simulink model "nmsRR"  (R2021a)
settings: Solver=ode15s  StartTime=0.0  StopTime=t  MaxStep=1e-2  RelTol=1e-2
StartFcn:
  | tic
StopFcn:
  | toc
  | 
  | 
  | %if GimbalLockFlag
  |  % fprintf(2, 'Almost reached Gimbal Lock of IMU. Simulation stopped.\n')
  | %end
  | 
  | %fprintf('Elapsed time: %4.2f sec (%4.2f%% realtime)\n', a, tout(end)/a*100)
undefined symbols (not defined in the file): Balance02, Balance13, BalanceTrunk, BasisStim, CompensateSwing, CompliantLeg, FlexAnkle, Ground, ICs, init_des_left, init_des_right, init_l_left, init_l_right, init_q_del, init_sensor_body, init_sensor_world, init_v_left, init_v_right, LateralControl, mParams, PreventKneeOverextension, StepDur, Target02, Target13, theta0, X, Y, Z
libraries: simulink_extras x133, nesl_utility x105, sm_lib x88, simulink x72, robotcorelib x5, dspinverses x5, dspswit3 x2, vrlib x2, robotmaniplib x1
(part 7 of 8)

== system nmsRR/Body and Contact Model/Vestibular System/Align Axis/Compute Saggital Rotation ==
  Hip Position Left [m] : Inport
  Hip Position Right [m] : Inport  Port=2
  Trunk Position [m] : Inport  Port=3
  Constant : Constant  Value=[0 1 0]
  Constant1 : Constant
  Constant2 : Constant  Value=-1
  Dot Product : DotProduct  InputSameDT=on  OutDataTypeStr=Inherit: Inherit via internal rule
  Gain : Gain  Gain=[0.5 0.5 0]
  Gain1 : Gain  Gain=[1 1 0]
  Minus : Sum
  Minus1 : Sum  Inputs=+-
  Product : Product
  Selector : Selector  InputPortWidth=3  IndexOptions=Index vector (dialog)  Indices=[1]  OutputSizes=1
  Switch : Switch  Criteria=u2 > Threshold
  Trigonometric Function : Trigonometry  Operator=acos
  compute angle witth y axis5 : Subsystem  Commented=on
  normalize : Subsystem
  Saggital Rotation : Outport
  wires:
  Hip Position Right [m]/1 -> Minus/1
  Trigonometric Function/1 -> Product/2
  Constant/1 -> Dot Product/1
  Dot Product/1 -> Trigonometric Function/1
  Hip Position Left [m]/1 -> Minus/2
  Minus/1 -> Gain/1
  Gain/1 -> Minus1/2
  Trunk Position [m]/1 -> Gain1/1
  Minus1/1 -> normalize/1(vector)
  Selector/1 -> Switch/2
  normalize/1(norm) -> compute angle witth y axis5/1(vector), Dot Product/2, Selector/1
  Constant1/1 -> Switch/3
  Constant2/1 -> Switch/1
  Switch/1 -> Product/1
  Product/1 -> Saggital Rotation/1
  Gain1/1 -> Minus1/1

== system nmsRR/Body and Contact Model/Vestibular System/R Movement direction/normalize ==
  vector : Inport
  Divide : Product  Inputs=*/  RndMeth=Zero  SaturateOnIntegerOverflow=on
  Matrix Sum : Sum  Inputs=+
  Sqrt : Sqrt  SaturateOnIntegerOverflow=on
  Square : Math  Operator=square  SaturateOnIntegerOverflow=on
  norm : Outport
  wires:
  vector/1 -> Square/1, Divide/1
  Matrix Sum/1 -> Sqrt/1
  Divide/1 -> norm/1
  Sqrt/1 -> Divide/2
  Square/1 -> Matrix Sum/1

== system nmsRR/Muscle Actuation Layer/Muscles Left/Muscle Dynamics (Vectorized)1/BE force-length relation ==
  note: Buffer Elasticity BE
  lce [lopt] : Inport
  Constant1 : Constant  Value=1-mParams.muscles.w
  Math Function : Math  Operator=square  SignedPower=on  SaturateOnIntegerOverflow=on
  Sum4 : Sum  Inputs=|+-  InputSameDT=on  SaturateOnIntegerOverflow=on  OutDataTypeStr=Inherit: Same as first input
  buffer engaged? : simulink/Logic and Bit Operations/Compare To Zero  relop=<  OutDataTypeStr=boolean  ZeroCross=off
  force of buffer elasticity : Product  Inputs=**
  reference strain [lslack] : Constant  Value=mParams.muscles.w/2
  relative strain : Product  Inputs=*/
  fbe [Fmax] : Outport  VectorParamsAs1DForOutWhenUnconnected=off
  wires:
  force of buffer elasticity/1 -> fbe [Fmax]/1
  Math Function/1 -> force of buffer elasticity/2
  buffer engaged?/1 -> force of buffer elasticity/1
  Constant1/1 -> Sum4/2
  Sum4/1 -> relative strain/1, buffer engaged?/1
  reference strain [lslack]/1 -> relative strain/2
  relative strain/1 -> Math Function/1
  lce [lopt]/1 -> Sum4/1

== system nmsRR/Muscle Actuation Layer/Muscles Left/Muscle Dynamics (Vectorized)1/CE force-length relation ==
  note: CE Force-Length Relationship
  lce [lopt] : Inport
  Abs : Abs
  Constant1 : Constant
  Constant2 : Constant  Value=3
  Gain : Gain  Gain=log(mParams.muscles.c)
  Math Function : Math  SignedPower=on  SaturateOnIntegerOverflow=on
  Math Function1 : Math  Operator=pow  SignedPower=on  SaturateOnIntegerOverflow=on
  Sum4 : Sum  Inputs=|+-  InputSameDT=on  SaturateOnIntegerOverflow=on  OutDataTypeStr=Inherit: Same as first input
  normalized position : Product  Inputs=*/
  relative width : Constant  Value=mParams.muscles.w
  fce [Fmax] : Outport  VectorParamsAs1DForOutWhenUnconnected=off
  wires:
  Math Function/1 -> fce [Fmax]/1
  Gain/1 -> Math Function/1
  Math Function1/1 -> Gain/1
  Constant2/1 -> Math Function1/2
  normalized position/1 -> Math Function1/1
  Abs/1 -> normalized position/1
  Sum4/1 -> Abs/1
  Constant1/1 -> Sum4/2
  relative width/1 -> normalized position/2
  lce [lopt]/1 -> Sum4/1

== system nmsRR/Muscle Actuation Layer/Muscles Left/Muscle Dynamics (Vectorized)1/CE inverse force-velocity relation ==
  note: CE Inverse Force-Velocity Relationship
  Fv[Fmax] : Inport
  1 : Product  Inputs=/*
  Constant{1,3..4,8} (4 alike) : Constant
  Constant2 : Constant  Value=mParams.muscles.N
  Curvature : Gain  Gain=mParams.muscles.K  SaturateOnIntegerOverflow=on  OutDataTypeStr=Inherit: Same as input  ParamDataTypeStr=Inherit: Same as input
  Curvature1 : Gain  Gain=7.56*mParams.muscles.K  SaturateOnIntegerOverflow=on  OutDataTypeStr=Inherit: Same as input  ParamDataTypeStr=Inherit: Same as input
  Logical Operator : Logic  Operator=NOT  AllPortsSameDT=off  OutDataTypeStr=boolean
  Logical Operator1 : Logic  Operator=NOT  AllPortsSameDT=off  OutDataTypeStr=boolean
  Slope : Gain  Gain=1e-2  SaturateOnIntegerOverflow=on  OutDataTypeStr=Inherit: Same as input  ParamDataTypeStr=Inherit: Same as input
  Sum1 : Sum  Inputs=|++  InputSameDT=on  SaturateOnIntegerOverflow=on  OutDataTypeStr=Inherit: Same as first input
  Sum2 : Sum  InputSameDT=on  SaturateOnIntegerOverflow=on  OutDataTypeStr=Inherit: Same as first input
  Sum3 : Sum  Inputs=++|  InputSameDT=on  SaturateOnIntegerOverflow=on  OutDataTypeStr=Inherit: Same as first input
  Sum4 : Sum  Inputs=|+-  InputSameDT=on  SaturateOnIntegerOverflow=on  OutDataTypeStr=Inherit: Same as first input
  Sum5 : Sum  Inputs=|-+  InputSameDT=on  SaturateOnIntegerOverflow=on  OutDataTypeStr=Inherit: Same as first input
  Sum6 : Sum  Inputs=-+|  InputSameDT=on  SaturateOnIntegerOverflow=on  OutDataTypeStr=Inherit: Same as first input
  Sum7 : Sum  Inputs=|++  InputSameDT=on  SaturateOnIntegerOverflow=on  OutDataTypeStr=Inherit: Same as first input
  Sum8 : Sum  Inputs=+-|  InputSameDT=on  SaturateOnIntegerOverflow=on  OutDataTypeStr=Inherit: Same as first input
  Sum9 : Sum  InputSameDT=on  SaturateOnIntegerOverflow=on  OutDataTypeStr=Inherit: Same as first input
  extension force within bound? : simulink/Logic and Bit Operations/Compare To Constant  relop=<=  const=mParams.muscles.N  OutDataTypeStr=boolean  ZeroCross=off
  force indicating contraction? : simulink/Logic and Bit Operations/Compare To Constant  relop=<=  const=1  OutDataTypeStr=boolean  ZeroCross=off
  v_concentric : Product  Inputs=*/
  v_concentric1 : Product  Inputs=**
  v_excentric <=N 1 : Product  Inputs=***
  v_excentric <N : Product  Inputs=*/
  v_excentric >N : Product  Inputs=**
  v[vmax] : Outport  VectorParamsAs1DForOutWhenUnconnected=off
  wires:
  Sum2/1 -> Sum9/2
  v_excentric <=N 1/1 -> Sum2/1
  Logical Operator1/1 -> v_excentric >N/1
  v_excentric >N/1 -> Sum2/2
  Logical Operator/1 -> v_excentric <=N 1/1
  Fv[Fmax]/1 -> extension force within bound?/1, force indicating contraction?/1, Curvature/1, Sum4/1, Sum6/2
  extension force within bound?/1 -> Logical Operator1/1, v_excentric <=N 1/3
  force indicating contraction?/1 -> Logical Operator/1, v_concentric1/2
  Sum1/1 -> v_excentric >N/2
  v_concentric1/1 -> Sum9/1
  v_excentric <N/1 -> v_excentric <=N 1/2
  Constant3/1 -> Sum5/1
  Sum5/1 -> 1/1
  Constant2/1 -> Sum5/2, Sum6/1
  Sum6/1 -> Slope/1, 1/2
  Constant8/1 -> Sum1/2
  Slope/1 -> Sum1/1
  Sum9/1 -> v[vmax]/1
  v_concentric/1 -> v_concentric1/1
  Sum7/1 -> v_excentric <N/1
  Sum8/1 -> v_excentric <N/2
  Curvature1/1 -> Sum8/2
  Constant4/1 -> Sum8/1, Sum7/2
  1/1 -> Curvature1/1, Sum7/1
  Sum3/1 -> v_concentric/2
  Sum4/1 -> v_concentric/1
  Constant1/1 -> Sum3/1, Sum4/2
  Curvature/1 -> Sum3/2

== system nmsRR/Muscle Actuation Layer/Muscles Left/Muscle Dynamics (Vectorized)1/PE force-length relation ==
  note: Parallel Elasticity PE
  lce [lopt] : Inport
  Constant3 : Constant
  Math Function2 : Math  Operator=square  SignedPower=on  SaturateOnIntegerOverflow=on
  Scope : Scope
  Scope1 : Scope
  Sum1 : Sum  Inputs=|+-  InputSameDT=on  SaturateOnIntegerOverflow=on  OutDataTypeStr=Inherit: Same as first input
  force of buffer elasticity : Product  Inputs=**
  parallel elasticity engaged? : simulink/Logic and Bit Operations/Compare To Zero  relop=>  OutDataTypeStr=boolean  ZeroCross=off
  reference strain [lopt] : Constant  Value=mParams.muscles.w
  relative strain : Product  Inputs=*/
  fpe [Fmax] : Outport  VectorParamsAs1DForOutWhenUnconnected=off
  wires:
  parallel elasticity engaged?/1 -> force of buffer elasticity/1
  force of buffer elasticity/1 -> fpe [Fmax]/1
  Math Function2/1 -> force of buffer elasticity/2
  relative strain/1 -> Math Function2/1
  reference strain [lopt]/1 -> relative strain/2
  Sum1/1 -> Scope/1, relative strain/1, parallel elasticity engaged?/1
  Constant3/1 -> Sum1/2
  lce [lopt]/1 -> Scope1/1, Sum1/1

== system nmsRR/Muscle Actuation Layer/Muscles Left/Muscle Dynamics (Vectorized)1/SE force-length relation ==
  note: SE Force-Length Relationship
  lse [lslack] : Inport
  Constant1 : Constant
  Math Function : Math  Operator=square  SignedPower=on  SaturateOnIntegerOverflow=on
  Scope : Scope
  Sum4 : Sum  Inputs=|+-  InputSameDT=on  SaturateOnIntegerOverflow=on  OutDataTypeStr=Inherit: Same as first input
  force above slack length : Product  Inputs=**
  greater than slack length? : simulink/Logic and Bit Operations/Compare To Zero  relop=>  OutDataTypeStr=boolean  ZeroCross=off
  reference strain [lslack] : Constant  Value=mParams.muscles.eref
  relative strain : Product  Inputs=*/
  fse [Fmax] : Outport  VectorParamsAs1DForOutWhenUnconnected=off
  wires:
  force above slack length/1 -> fse [Fmax]/1
  greater than slack length?/1 -> Scope/1, force above slack length/1
  Sum4/1 -> relative strain/1, greater than slack length?/1
  reference strain [lslack]/1 -> relative strain/2
  relative strain/1 -> Math Function/1
  lse [lslack]/1 -> Sum4/1
  Math Function/1 -> force above slack length/2
  Constant1/1 -> Sum4/2

== system nmsRR/Muscle Actuation Layer/Muscles Right/Muscle Dynamics (Vectorized)/BE force-length relation ==
  note: Buffer Elasticity BE
  lce [lopt] : Inport
  Constant1 : Constant  Value=1-mParams.muscles.w
  Math Function : Math  Operator=square  SignedPower=on  SaturateOnIntegerOverflow=on
  Sum4 : Sum  Inputs=|+-  InputSameDT=on  SaturateOnIntegerOverflow=on  OutDataTypeStr=Inherit: Same as first input
  buffer engaged? : simulink/Logic and Bit Operations/Compare To Zero  relop=<  OutDataTypeStr=boolean  ZeroCross=off
  force of buffer elasticity : Product  Inputs=**
  reference strain [lslack] : Constant  Value=mParams.muscles.w/2
  relative strain : Product  Inputs=*/
  fbe [Fmax] : Outport  VectorParamsAs1DForOutWhenUnconnected=off
  wires:
  force of buffer elasticity/1 -> fbe [Fmax]/1
  Math Function/1 -> force of buffer elasticity/2
  buffer engaged?/1 -> force of buffer elasticity/1
  Constant1/1 -> Sum4/2
  Sum4/1 -> relative strain/1, buffer engaged?/1
  reference strain [lslack]/1 -> relative strain/2
  relative strain/1 -> Math Function/1
  lce [lopt]/1 -> Sum4/1

== system nmsRR/Muscle Actuation Layer/Muscles Right/Muscle Dynamics (Vectorized)/CE force-length relation ==
  note: CE Force-Length Relationship
  lce [lopt] : Inport
  Abs : Abs
  Constant1 : Constant
  Constant2 : Constant  Value=3
  Gain : Gain  Gain=log(mParams.muscles.c)
  Math Function : Math  SignedPower=on  SaturateOnIntegerOverflow=on
  Math Function1 : Math  Operator=pow  SignedPower=on  SaturateOnIntegerOverflow=on
  Sum4 : Sum  Inputs=|+-  InputSameDT=on  SaturateOnIntegerOverflow=on  OutDataTypeStr=Inherit: Same as first input
  normalized position : Product  Inputs=*/
  relative width : Constant  Value=mParams.muscles.w
  fce [Fmax] : Outport  VectorParamsAs1DForOutWhenUnconnected=off
  wires:
  Math Function/1 -> fce [Fmax]/1
  Gain/1 -> Math Function/1
  Math Function1/1 -> Gain/1
  Constant2/1 -> Math Function1/2
  normalized position/1 -> Math Function1/1
  Abs/1 -> normalized position/1
  Sum4/1 -> Abs/1
  Constant1/1 -> Sum4/2
  relative width/1 -> normalized position/2
  lce [lopt]/1 -> Sum4/1

== system nmsRR/Muscle Actuation Layer/Muscles Right/Muscle Dynamics (Vectorized)/CE inverse force-velocity relation ==
  note: CE Inverse Force-Velocity Relationship
  Fv[Fmax] : Inport
  1 : Product  Inputs=/*
  Constant{1,3..4,8} (4 alike) : Constant
  Constant2 : Constant  Value=mParams.muscles.N
  Curvature : Gain  Gain=mParams.muscles.K  SaturateOnIntegerOverflow=on  OutDataTypeStr=Inherit: Same as input  ParamDataTypeStr=Inherit: Same as input
  Curvature1 : Gain  Gain=7.56*mParams.muscles.K  SaturateOnIntegerOverflow=on  OutDataTypeStr=Inherit: Same as input  ParamDataTypeStr=Inherit: Same as input
  Logical Operator : Logic  Operator=NOT  AllPortsSameDT=off  OutDataTypeStr=boolean
  Logical Operator1 : Logic  Operator=NOT  AllPortsSameDT=off  OutDataTypeStr=boolean
  Slope : Gain  Gain=1e-2  SaturateOnIntegerOverflow=on  OutDataTypeStr=Inherit: Same as input  ParamDataTypeStr=Inherit: Same as input
  Sum1 : Sum  Inputs=|++  InputSameDT=on  SaturateOnIntegerOverflow=on  OutDataTypeStr=Inherit: Same as first input
  Sum2 : Sum  InputSameDT=on  SaturateOnIntegerOverflow=on  OutDataTypeStr=Inherit: Same as first input
  Sum3 : Sum  Inputs=++|  InputSameDT=on  SaturateOnIntegerOverflow=on  OutDataTypeStr=Inherit: Same as first input
  Sum4 : Sum  Inputs=|+-  InputSameDT=on  SaturateOnIntegerOverflow=on  OutDataTypeStr=Inherit: Same as first input
  Sum5 : Sum  Inputs=|-+  InputSameDT=on  SaturateOnIntegerOverflow=on  OutDataTypeStr=Inherit: Same as first input
  Sum6 : Sum  Inputs=-+|  InputSameDT=on  SaturateOnIntegerOverflow=on  OutDataTypeStr=Inherit: Same as first input
  Sum7 : Sum  Inputs=|++  InputSameDT=on  SaturateOnIntegerOverflow=on  OutDataTypeStr=Inherit: Same as first input
  Sum8 : Sum  Inputs=+-|  InputSameDT=on  SaturateOnIntegerOverflow=on  OutDataTypeStr=Inherit: Same as first input
  Sum9 : Sum  InputSameDT=on  SaturateOnIntegerOverflow=on  OutDataTypeStr=Inherit: Same as first input
  extension force within bound? : simulink/Logic and Bit Operations/Compare To Constant  relop=<=  const=mParams.muscles.N  OutDataTypeStr=boolean  ZeroCross=off
  force indicating contraction? : simulink/Logic and Bit Operations/Compare To Constant  relop=<=  const=1  OutDataTypeStr=boolean  ZeroCross=off
  v_concentric : Product  Inputs=*/
  v_concentric1 : Product  Inputs=**
  v_excentric <=N 1 : Product  Inputs=***
  v_excentric <N : Product  Inputs=*/
  v_excentric >N : Product  Inputs=**
  v[vmax] : Outport  VectorParamsAs1DForOutWhenUnconnected=off
  wires:
  Sum2/1 -> Sum9/2
  v_excentric <=N 1/1 -> Sum2/1
  Logical Operator1/1 -> v_excentric >N/1
  v_excentric >N/1 -> Sum2/2
  Logical Operator/1 -> v_excentric <=N 1/1
  Fv[Fmax]/1 -> extension force within bound?/1, force indicating contraction?/1, Curvature/1, Sum4/1, Sum6/2
  extension force within bound?/1 -> Logical Operator1/1, v_excentric <=N 1/3
  force indicating contraction?/1 -> Logical Operator/1, v_concentric1/2
  Sum1/1 -> v_excentric >N/2
  v_concentric1/1 -> Sum9/1
  v_excentric <N/1 -> v_excentric <=N 1/2
  Constant3/1 -> Sum5/1
  Sum5/1 -> 1/1
  Constant2/1 -> Sum5/2, Sum6/1
  Sum6/1 -> Slope/1, 1/2
  Constant8/1 -> Sum1/2
  Slope/1 -> Sum1/1
  Sum9/1 -> v[vmax]/1
  v_concentric/1 -> v_concentric1/1
  Sum7/1 -> v_excentric <N/1
  Sum8/1 -> v_excentric <N/2
  Curvature1/1 -> Sum8/2
  Constant4/1 -> Sum8/1, Sum7/2
  1/1 -> Curvature1/1, Sum7/1
  Sum3/1 -> v_concentric/2
  Sum4/1 -> v_concentric/1
  Constant1/1 -> Sum3/1, Sum4/2
  Curvature/1 -> Sum3/2

== system nmsRR/Muscle Actuation Layer/Muscles Right/Muscle Dynamics (Vectorized)/PE force-length relation ==
  note: Parallel Elasticity PE
  lce [lopt] : Inport
  Constant3 : Constant
  Math Function2 : Math  Operator=square  SignedPower=on  SaturateOnIntegerOverflow=on
  Sum1 : Sum  Inputs=|+-  InputSameDT=on  SaturateOnIntegerOverflow=on  OutDataTypeStr=Inherit: Same as first input
  force of buffer elasticity : Product  Inputs=**
  parallel elasticity engaged? : simulink/Logic and Bit Operations/Compare To Zero  relop=>  OutDataTypeStr=boolean  ZeroCross=off
  reference strain [lopt] : Constant  Value=mParams.muscles.w
  relative strain : Product  Inputs=*/
  fpe [Fmax] : Outport  VectorParamsAs1DForOutWhenUnconnected=off
  wires:
  parallel elasticity engaged?/1 -> force of buffer elasticity/1
  force of buffer elasticity/1 -> fpe [Fmax]/1
  Math Function2/1 -> force of buffer elasticity/2
  relative strain/1 -> Math Function2/1
  reference strain [lopt]/1 -> relative strain/2
  Sum1/1 -> relative strain/1, parallel elasticity engaged?/1
  Constant3/1 -> Sum1/2
  lce [lopt]/1 -> Sum1/1

== system nmsRR/Muscle Actuation Layer/Muscles Right/Muscle Dynamics (Vectorized)/SE force-length relation ==
  note: SE Force-Length Relationship
  lse [lslack] : Inport
  Constant1 : Constant
  Math Function : Math  Operator=square  SignedPower=on  SaturateOnIntegerOverflow=on
  Scope{,1..3} (4 alike) : Scope
  Selector : Selector  InputPortWidth=11  IndexOptions=Index vector (dialog)  Indices=[1]  OutputSizes=1
  Sum4 : Sum  Inputs=|+-  InputSameDT=on  SaturateOnIntegerOverflow=on  OutDataTypeStr=Inherit: Same as first input
  force above slack length : Product  Inputs=**
  greater than slack length? : simulink/Logic and Bit Operations/Compare To Zero  relop=>  OutDataTypeStr=boolean  ZeroCross=off
  reference strain [lslack] : Constant  Value=mParams.muscles.eref
  relative strain : Product  Inputs=*/
  fse [Fmax] : Outport  VectorParamsAs1DForOutWhenUnconnected=off
  wires:
  force above slack length/1 -> Scope1/1, fse [Fmax]/1
  greater than slack length?/1 -> Scope2/1, force above slack length/1
  Constant1/1 -> Sum4/2
  Sum4/1 -> relative strain/1, greater than slack length?/1
  relative strain/1 -> Math Function/1
  lse [lslack]/1 -> Selector/1, Sum4/1
  Math Function/1 -> Scope3/1, force above slack length/2
  reference strain [lslack]/1 -> relative strain/2
  Selector/1 -> Scope/1

== system nmsRR/Supraspinal Level/Subsystem/Compute Acceleration Profiles with Minimal Jerk Approach/ Timer Phase 1 ==
  R : Inport
  Clock1 : Clock
  Clock3 : Clock
      settings: Decimation=4
  NOT : Logic  Operator=NOT  AllPortsSameDT=off  OutDataTypeStr=boolean
  Resettable Subsystem : Subsystem  TreatAsAtomicUnit=on
  Sum1 : Sum  Inputs=|+-  InputSameDT=on  SaturateOnIntegerOverflow=on  OutDataTypeStr=Inherit: Same as first input
  Switch2 : Switch  Criteria=u2 > Threshold  RndMeth=Zero  ZeroCross=off
  Out : Outport  VectorParamsAs1DForOutWhenUnconnected=off
  wires:
  Clock1/1 -> Sum1/1
  Clock3/1 -> Switch2/3, Resettable Subsystem/1(In1)
  Sum1/1 -> Out/1
  R/1 -> NOT/1, Switch2/2
  Switch2/1 -> Sum1/2
  Resettable Subsystem/1(Out1) -> Switch2/1
  NOT/1 -> Resettable Subsystem/Enable

== system nmsRR/Supraspinal Level/Subsystem/Compute Acceleration Profiles with Minimal Jerk Approach/ Timer Phase 2 ==
  R : Inport
  Clock1 : Clock
  Clock3 : Clock
      settings: Decimation=4
  NOT : Logic  Operator=NOT  AllPortsSameDT=off  OutDataTypeStr=boolean
  Resettable Subsystem : Subsystem  TreatAsAtomicUnit=on
  Sum1 : Sum  Inputs=|+-  InputSameDT=on  SaturateOnIntegerOverflow=on  OutDataTypeStr=Inherit: Same as first input
  Switch2 : Switch  Criteria=u2 > Threshold  RndMeth=Zero  ZeroCross=off
  Out : Outport  VectorParamsAs1DForOutWhenUnconnected=off
  wires:
  Clock1/1 -> Sum1/1
  Clock3/1 -> Switch2/3, Resettable Subsystem/1(In1)
  Sum1/1 -> Out/1
  R/1 -> NOT/1, Switch2/2
  Switch2/1 -> Sum1/2
  Resettable Subsystem/1(Out1) -> Switch2/1
  NOT/1 -> Resettable Subsystem/Enable

== system nmsRR/Supraspinal Level/Subsystem/Compute Acceleration Profiles with Minimal Jerk Approach/Minimal jerk Hip Pitch1 ==
  T_tot : Inport
  t_passed : Inport  Port=2
  "x0, dx0, ddx0" : Inport  Port=3
  "xT, dxT, ddxT" : Inport  Port=4
  Compare To Constant : simulink/Logic and Bit Operations/Compare To Constant  relop=>=  const=mParams.control.timelimit  OutDataTypeStr=boolean  ZeroCross=off
  Constant : Constant  Value=mParams.control.timelimit
  Constant1 : Constant  Value=0
  Demux : Demux  Outputs=3
  Demux1 : Demux  Outputs=3
  Enabled Subsystem : Subsystem  TreatAsAtomicUnit=on
  Minimal Jerk : Subsystem
  Minimal Jerk Parameters [Movellan] : Subsystem
  Minus : Sum  Inputs=+-
  Minus1 : Sum  Inputs=+-
  Switch : Switch  Criteria=u2 ~= 0  ZeroCross=off
  jerk : Outport
  wires:
  Minimal Jerk/1(j(t)) -> jerk/1
  T_tot/1 -> Minus/1
  t_passed/1 -> Minus/2
  Constant1/1 -> Switch/1
  Demux/1 -> Minimal Jerk Parameters [Movellan]/1(x0)
  Demux/2 -> Minimal Jerk Parameters [Movellan]/2(dx0)
  Demux/3 -> Minimal Jerk Parameters [Movellan]/3(ddx0)
  Demux1/1 -> Minimal Jerk Parameters [Movellan]/4(xT)
  "x0, dx0, ddx0"/1 -> Demux/1
  Demux1/2 -> Minimal Jerk Parameters [Movellan]/5(dxT)
  "xT, dxT, ddxT"/1 -> Demux1/1
  Demux1/3 -> Minimal Jerk Parameters [Movellan]/6(ddxT)
  Minimal Jerk Parameters [Movellan]/1(a) -> Enabled Subsystem/1(In1)
  Minus/1 -> Compare To Constant/1, Minus1/2, Minimal Jerk Parameters [Movellan]/7(T)
  Enabled Subsystem/1(Out1) -> Minimal Jerk/2(a [6x1])
  Compare To Constant/1 -> Switch/2, Enabled Subsystem/Enable
  Constant/1 -> Minus1/1
  Minus1/1 -> Switch/3
  Switch/1 -> Minimal Jerk/1(t)

== system nmsRR/Supraspinal Level/Subsystem/Compute Acceleration Profiles with Minimal Jerk Approach/Minimal jerk Hip Pitch2 ==
  T_tot : Inport
  t_passed : Inport  Port=2
  "x0, dx0, ddx0" : Inport  Port=3
  "xT, dxT, ddxT" : Inport  Port=4
  Compare To Constant : simulink/Logic and Bit Operations/Compare To Constant  relop=>=  const=mParams.control.timelimit  OutDataTypeStr=boolean  ZeroCross=off
  Constant : Constant  Value=mParams.control.timelimit
  Constant1 : Constant  Value=0
  Demux : Demux  Outputs=3
  Demux1 : Demux  Outputs=3
  Enabled Subsystem : Subsystem  TreatAsAtomicUnit=on
  Minimal Jerk : Subsystem
  Minimal Jerk Parameters [Movellan] : Subsystem
  Minus : Sum  Inputs=+-
  Minus1 : Sum  Inputs=+-
  Switch : Switch  Criteria=u2 ~= 0  ZeroCross=off
  jerk : Outport
  wires:
  Minimal Jerk/1(j(t)) -> jerk/1
  T_tot/1 -> Minus/1
  t_passed/1 -> Minus/2
  Constant1/1 -> Switch/1
  Demux/1 -> Minimal Jerk Parameters [Movellan]/1(x0)
  Demux/2 -> Minimal Jerk Parameters [Movellan]/2(dx0)
  Demux/3 -> Minimal Jerk Parameters [Movellan]/3(ddx0)
  Demux1/1 -> Minimal Jerk Parameters [Movellan]/4(xT)
  "x0, dx0, ddx0"/1 -> Demux/1
  Demux1/2 -> Minimal Jerk Parameters [Movellan]/5(dxT)
  "xT, dxT, ddxT"/1 -> Demux1/1
  Demux1/3 -> Minimal Jerk Parameters [Movellan]/6(ddxT)
  Minimal Jerk Parameters [Movellan]/1(a) -> Enabled Subsystem/1(In1)
  Minus/1 -> Compare To Constant/1, Minus1/2, Minimal Jerk Parameters [Movellan]/7(T)
  Enabled Subsystem/1(Out1) -> Minimal Jerk/2(a [6x1])
  Compare To Constant/1 -> Switch/2, Enabled Subsystem/Enable
  Constant/1 -> Minus1/1
  Minus1/1 -> Switch/3
  Switch/1 -> Minimal Jerk/1(t)

== system nmsRR/Supraspinal Level/Subsystem/Compute Acceleration Profiles with Minimal Jerk Approach/Minimal jerk Hip Pitch3 ==
  T_tot : Inport
  t_passed : Inport  Port=2
  "x0, dx0, ddx0" : Inport  Port=3
  "xT, dxT, ddxT" : Inport  Port=4
  Compare To Constant1 : simulink/Logic and Bit Operations/Compare To Constant  relop=>=  const=mParams.control.timelimit  OutDataTypeStr=boolean  ZeroCross=off
  Constant : Constant  Value=mParams.control.timelimit
  Constant1 : Constant  Value=0
  Demux : Demux  Outputs=3
  Demux1 : Demux  Outputs=3
  Enabled Subsystem : Subsystem  TreatAsAtomicUnit=on
  Minimal Jerk : Subsystem
  Minimal Jerk Parameters [Movellan] : Subsystem
  Minus : Sum  Inputs=+-
  Minus1 : Sum  Inputs=+-
  Switch : Switch  Criteria=u2 ~= 0  ZeroCross=off
  jerk : Outport
  wires:
  Minimal Jerk/1(j(t)) -> jerk/1
  T_tot/1 -> Minus/1
  t_passed/1 -> Minus/2
  Constant1/1 -> Switch/1
  Demux/1 -> Minimal Jerk Parameters [Movellan]/1(x0)
  Demux/2 -> Minimal Jerk Parameters [Movellan]/2(dx0)
  Demux/3 -> Minimal Jerk Parameters [Movellan]/3(ddx0)
  Demux1/1 -> Minimal Jerk Parameters [Movellan]/4(xT)
  "x0, dx0, ddx0"/1 -> Demux/1
  Demux1/2 -> Minimal Jerk Parameters [Movellan]/5(dxT)
  "xT, dxT, ddxT"/1 -> Demux1/1
  Demux1/3 -> Minimal Jerk Parameters [Movellan]/6(ddxT)
  Minimal Jerk Parameters [Movellan]/1(a) -> Enabled Subsystem/1(In1)
  Minus/1 -> Compare To Constant1/1, Minus1/2, Minimal Jerk Parameters [Movellan]/7(T)
  Enabled Subsystem/1(Out1) -> Minimal Jerk/2(a [6x1])
  Compare To Constant1/1 -> Switch/2, Enabled Subsystem/Enable
  Constant/1 -> Minus1/1
  Minus1/1 -> Switch/3
  Switch/1 -> Minimal Jerk/1(t)

== system nmsRR/Supraspinal Level/Subsystem/Compute Acceleration Profiles with Minimal Jerk Approach/Minimal jerk Hip Pitch4 ==
  T_tot : Inport
  t_passed : Inport  Port=2
  "x0, dx0, ddx0" : Inport  Port=3
  "xT, dxT, ddxT" : Inport  Port=4
  Compare To Constant : simulink/Logic and Bit Operations/Compare To Constant  relop=>=  const=mParams.control.timelimit  OutDataTypeStr=boolean  ZeroCross=off
  Constant : Constant  Value=mParams.control.timelimit
  Constant1 : Constant  Value=0
  Demux : Demux  Outputs=3
  Demux1 : Demux  Outputs=3
  Enabled Subsystem : Subsystem  TreatAsAtomicUnit=on
  Minimal Jerk : Subsystem
  Minimal Jerk Parameters [Movellan] : Subsystem
  Minus : Sum  Inputs=+-
  Minus1 : Sum  Inputs=+-
  Switch : Switch  Criteria=u2 ~= 0  ZeroCross=off
  jerk : Outport
  wires:
  Minimal Jerk/1(j(t)) -> jerk/1
  T_tot/1 -> Minus/1
  t_passed/1 -> Minus/2
  Constant1/1 -> Switch/1
  Demux/1 -> Minimal Jerk Parameters [Movellan]/1(x0)
  Demux/2 -> Minimal Jerk Parameters [Movellan]/2(dx0)
  Demux/3 -> Minimal Jerk Parameters [Movellan]/3(ddx0)
  Demux1/1 -> Minimal Jerk Parameters [Movellan]/4(xT)
  "x0, dx0, ddx0"/1 -> Demux/1
  Demux1/2 -> Minimal Jerk Parameters [Movellan]/5(dxT)
  "xT, dxT, ddxT"/1 -> Demux1/1
  Demux1/3 -> Minimal Jerk Parameters [Movellan]/6(ddxT)
  Minimal Jerk Parameters [Movellan]/1(a) -> Enabled Subsystem/1(In1)
  Minus/1 -> Compare To Constant/1, Minus1/2, Minimal Jerk Parameters [Movellan]/7(T)
  Enabled Subsystem/1(Out1) -> Minimal Jerk/2(a [6x1])
  Compare To Constant/1 -> Switch/2, Enabled Subsystem/Enable
  Constant/1 -> Minus1/1
  Minus1/1 -> Switch/3
  Switch/1 -> Minimal Jerk/1(t)

== system nmsRR/Supraspinal Level/Subsystem/Compute Target States/Balance Control lateral ==
  Left/Right : Inport
  Constant : Constant  Value=0
  Divide : Product  Inputs=**
  Divide1 : Product  Inputs=**
  Minus5 : Sum  Inputs=+++
  Minus6 : Sum  Inputs=+-
  Selector3 : Selector  InputPortWidth=3  IndexOptions=Index vector (dialog)  Indices=[3]  OutputSizes=1
  Selector4 : Selector  InputPortWidth=3  IndexOptions=Index vector (dialog)  Indices=[3]  OutputSizes=1
  Selector5 : Selector  InputPortWidth=3  IndexOptions=Index vector (dialog)  Indices=[3]  OutputSizes=1
  Switch : Switch  Criteria=u2 > Threshold
  theta_Hip_swing_target : Outport
  wires:
  Divide/1 -> Minus5/2
  [swh_lat] -> Minus5/1
  Switch/1 -> Minus6/2
  Divide1/1 -> Minus5/3
  [AnklePosR_rot] -> Selector3/1
  Minus6/1 -> Divide1/1
  Left/Right/1 -> Switch/2
  [AnklePosL_rot] -> Selector4/1
  [cv_lat] -> Divide/2
  [cd_lat] -> Divide1/2
  Selector4/1 -> Switch/1
  Selector3/1 -> Switch/3
  [CoM_Velocity_rot] -> Selector5/1
  Selector5/1 -> Divide/1
  Constant/1 -> Minus6/1
  Minus5/1 -> theta_Hip_swing_target/1

== system nmsRR/Supraspinal Level/Subsystem/Compute Target States/Balance Control saggital ==
  Left/Right : Inport
  Constant : Constant  Value=0
  Divide : Product  Inputs=**
  Divide1 : Product  Inputs=**
  Minus5 : Sum  Inputs=+++
  Minus6 : Sum  Inputs=+-
  Selector3 : Selector  InputPortWidth=3  IndexOptions=Index vector (dialog)  Indices=[1]  OutputSizes=1
  Selector4 : Selector  InputPortWidth=3  IndexOptions=Index vector (dialog)  Indices=[1]  OutputSizes=1
  Selector5 : Selector  InputPortWidth=3  IndexOptions=Index vector (dialog)  Indices=[1]  OutputSizes=1
  Switch : Switch  Criteria=u2 > Threshold
  theta_Hip_swing_target : Outport
  wires:
  [swh] -> Minus5/1
  Switch/1 -> Minus6/2
  [AnklePosR_rot] -> Selector4/1
  Minus6/1 -> Divide1/1
  Left/Right/1 -> Switch/2
  [AnklePosL_rot] -> Selector3/1
  [cv] -> Divide/2
  [cd] -> Divide1/2
  Selector3/1 -> Switch/1
  Selector4/1 -> Switch/3
  Divide/1 -> Minus5/2
  Divide1/1 -> Minus5/3
  [CoM_Velocity_rot] -> Selector5/1
  Selector5/1 -> Divide/1
  Constant/1 -> Minus6/1
  Minus5/1 -> theta_Hip_swing_target/1

== system nmsRR/Supraspinal Level/Subsystem/Inverse Dynamics/Inverse Dynamics ==
  note: Augment Joint Vectors: In order to compute appropriate gravitational and velocity dependend forces, the joint angle and joint angle acceleration vectors are augmented by the position and velocity of the body in space.
  Rotation Trunk [rad] : Inport
  Joint Angle Velocities [rad/s] : Inport  Port=2
  Joint Angles [rad] : Inport  Port=3
  Rotation Velocity Trunk [rad/s] : Inport  Port=4
  Trunk Position [m] : Inport  Port=5
  Trunk Velocity [m/s] : Inport  Port=6
  Desired Acceleration [rad/s^2] : Inport  Port=7
  Constant : Constant  Value=zeros(6,1)
  Inverse Dynamics : Subsystem
  Mux : Mux  Inputs=3
  Mux1 : Mux  Inputs=3
  Mux2 : Mux  Inputs=2
  " Desired Torques" : Outport  VectorParamsAs1DForOutWhenUnconnected=off
  wires:
  Trunk Position [m]/1 -> Mux1/1
  Inverse Dynamics/1(Desired Torques) -> " Desired Torques"/1
  Mux1/1 -> Inverse Dynamics/1(Config)
  Joint Angles [rad]/1 -> Mux1/3
  Rotation Trunk [rad]/1 -> Mux1/2
  Joint Angle Velocities [rad/s]/1 -> Mux/3
  Rotation Velocity Trunk [rad/s]/1 -> Mux/2
  Trunk Velocity [m/s]/1 -> Mux/1
  Mux/1 -> Inverse Dynamics/2(JointVel)
  Desired Acceleration [rad/s^2]/1 -> Mux2/2
  Constant/1 -> Mux2/1
  Mux2/1 -> Inverse Dynamics/3(JointAccel)

== system nmsRR/Supraspinal Level/Subsystem/Inverse Dynamics/Sensor Data from Body Layer ==
  " Rotation Trunk [rad]" : Outport
  Joint Angle Velocities [rad/s] : Outport  Port=2
  Joint Angles [rad] : Outport  Port=3
  Rotation Velocity Trunk [rad/s] : Outport  Port=4
  Trunk Position [m] : Outport  Port=5
  Trunk Velocity [m/s] : Outport  Port=6
  wires:
  [CoM_Position] -> Trunk Position [m]/1
  [RotationTrunk] -> " Rotation Trunk [rad]"/1
  [RotationVelocityTrunk] -> Rotation Velocity Trunk [rad/s]/1
  [q_delayed] -> Joint Angles [rad]/1
  [dq_delayed] -> Joint Angle Velocities [rad/s]/1
  [CoM_Velocity] -> Trunk Velocity [m/s]/1

== system nmsRR/Supraspinal Level/Subsystem/torques --> forces/F from T2 ==
  Desired Torques : Inport
  Matrix Multiply : Product  Multiplication=Matrix(*)
  Desired Forces : Outport
  wires:
  Desired Torques/1 -> Matrix Multiply/2
  Matrix Multiply/1 -> Desired Forces/1
  [C_transpose] -> Matrix Multiply/1

== system nmsRR/Supraspinal Level/Subsystem/torques --> forces/Moment Arm Matrix ==
  Lleg : Inport
  Rleg : Inport  Port=2
  Matrix Concatenate : Concatenate  NumInputs=8  Mode=Multidimensional array  ConcatenateDimension=2
  Row 1 : Subsystem
  Row 2 : Subsystem
  Row 3 : Subsystem
  Row 4 : Subsystem
  Row 5 : Subsystem
  Row 6 : Subsystem
  Row 7 : Subsystem
  Row 8 : Subsystem
  Selector : Selector  InputPortWidth=4  IndexOptions=Index vector (dialog)  Indices=[3]  OutputSizes=1
  Selector1 : Selector  InputPortWidth=4  IndexOptions=Index vector (dialog)  Indices=[4]  OutputSizes=1
  Selector2 : Selector  InputPortWidth=4  IndexOptions=Index vector (dialog)  Indices=[3]  OutputSizes=1
  Selector3 : Selector  InputPortWidth=4  IndexOptions=Index vector (dialog)  Indices=[4]  OutputSizes=1
  Moment Arm Matrix : Outport
  wires:
  Row 7/1(dl/theta7) -> Matrix Concatenate/7
  Row 8/1(dl/theta8) -> Matrix Concatenate/8
  Selector/1 -> Row 3/1(q(3))
  Row 5/1(dl/theta5) -> Matrix Concatenate/5
  Lleg/1 -> Selector1/1, Selector/1
  Selector2/1 -> Row 7/1(q(7))
  Row 2/1(dl/theta2) -> Matrix Concatenate/2
  Row 4/1(dl/theta4) -> Matrix Concatenate/4
  Row 3/1(dl/theta3) -> Matrix Concatenate/3
  Selector3/1 -> Row 8/1(q(8))
  Row 1/1(dl/theta1) -> Matrix Concatenate/1
  Rleg/1 -> Selector3/1, Selector2/1
  Selector1/1 -> Row 4/1(q(4))
  Row 6/1(dl/theta6) -> Matrix Concatenate/6
  Matrix Concatenate/1 -> Moment Arm Matrix/1

== system nmsRR/Supraspinal Level/Subsystem/torques --> forces/Separate Force ==
  Force : Inport
  Constant4 : Constant  Value=zeros(22,1)
  Max2 : MinMax  Function=max  Inputs=2  OutDataTypeStr=double  ZeroCross=off
  Max3 : MinMax  Inputs=2  OutDataTypeStr=double  ZeroCross=off
  Positive : Outport
  Negative : Outport  Port=2
  wires:
  Max3/1 -> Negative/1
  Max2/1 -> Positive/1
  Force/1 -> Max3/1, Max2/1
  Constant4/1 -> Max3/2, Max2/2

== system nmsRR/Supraspinal Level/Subsystem/torques --> forces/Subsystem1 ==
  Force : Inport
  F from T : Subsystem
  T from F : Subsystem
  separate Force : Subsystem
  Positive Part : Outport
  Negative Part : Outport  Port=2
  wires:
  Force/1 -> T from F/1(F)
  separate Force/1(Positive Part) -> Positive Part/1
  separate Force/2(Negative Part) -> Negative Part/1
  T from F/1(T) -> F from T/1(T)
  F from T/1(F) -> separate Force/1(Force)

== system nmsRR/Supraspinal Level/Subsystem/torques --> forces/Subsystem12 ==
  Force : Inport
  F from T : Subsystem
  T from F : Subsystem
  separate Force : Subsystem
  Positive Part : Outport
  Negative Part : Outport  Port=2
  wires:
  Force/1 -> T from F/1(F)
  separate Force/1(Positive Part) -> Positive Part/1
  separate Force/2(Negative Part) -> Negative Part/1
  T from F/1(T) -> F from T/1(T)
  F from T/1(F) -> separate Force/1(Force)

== system nmsRR/Supraspinal Level/Subsystem/torques --> forces/Subsystem2 ==
  Force : Inport
  F from T : Subsystem
  T from F : Subsystem
  separate Force : Subsystem
  Positive Part : Outport
  Negative Part : Outport  Port=2
  wires:
  Force/1 -> T from F/1(F)
  separate Force/1(Positive Part) -> Positive Part/1
  separate Force/2(Negative Part) -> Negative Part/1
  T from F/1(T) -> F from T/1(T)
  F from T/1(F) -> separate Force/1(Force)

== system nmsRR/Supraspinal Level/Subsystem/torques --> forces/Subsystem3 ==
  Force : Inport
  F from T : Subsystem
  T from F : Subsystem
  separate Force : Subsystem
  Positive Part : Outport
  Negative Part : Outport  Port=2
  wires:
  Force/1 -> T from F/1(F)
  separate Force/1(Positive Part) -> Positive Part/1
  separate Force/2(Negative Part) -> Negative Part/1
  T from F/1(T) -> F from T/1(T)
  F from T/1(F) -> separate Force/1(Force)

== system nmsRR/Supraspinal Level/Subsystem/torques --> forces/Subsystem4 ==
  Force : Inport
  F from T : Subsystem
  T from F : Subsystem
  separate Force : Subsystem
  Positive Part : Outport
  Negative Part : Outport  Port=2
  wires:
  Force/1 -> T from F/1(F)
  separate Force/1(Positive Part) -> Positive Part/1
  separate Force/2(Negative Part) -> Negative Part/1
  T from F/1(T) -> F from T/1(T)
  F from T/1(F) -> separate Force/1(Force)

== system nmsRR/Body and Contact Model/Vestibular System/Align Axis/Compute Lateral Rotation/normalize ==
  vector : Inport
  Divide : Product  Inputs=*/  RndMeth=Zero  SaturateOnIntegerOverflow=on
  Matrix Sum : Sum  Inputs=+
  Sqrt : Sqrt  SaturateOnIntegerOverflow=on
  Square : Math  Operator=square  SaturateOnIntegerOverflow=on
  norm : Outport
  wires:
  vector/1 -> Square/1, Divide/1
  Matrix Sum/1 -> Sqrt/1
  Divide/1 -> norm/1
  Sqrt/1 -> Divide/2
  Square/1 -> Matrix Sum/1

== system nmsRR/Body and Contact Model/Vestibular System/Align Axis/Compute Saggital Rotation/compute angle witth y axis5 ==
  vector : Inport
  Constant7 : Constant  Value=[0 1 0]
  Product : Product
  Rotation Between 2 Vectors : vrlib/Utilities/Rotation Between 2 Vectors
      settings: SourceProductBaseCode=SL
  Selector10 : Selector  InputPortWidth=4  IndexOptions=Index vector (dialog)  Indices=[1]  OutputSizes=1
  Selector9 : Selector  InputPortWidth=4  IndexOptions=Index vector (dialog)  Indices=[4]  OutputSizes=1
  angle [rad] : Outport
  wires:
  Product/1 -> angle [rad]/1
  vector/1 -> Rotation Between 2 Vectors/2
  Selector9/1 -> Product/1
  Constant7/1 -> Rotation Between 2 Vectors/1
  Rotation Between 2 Vectors/1 -> Selector9/1, Selector10/1
  Selector10/1 -> Product/2

== system nmsRR/Body and Contact Model/Vestibular System/Align Axis/Compute Saggital Rotation/normalize ==
  vector : Inport
  Divide : Product  Inputs=*/  RndMeth=Zero  SaturateOnIntegerOverflow=on
  Matrix Sum : Sum  Inputs=+
  Sqrt : Sqrt  SaturateOnIntegerOverflow=on
  Square : Math  Operator=square  SaturateOnIntegerOverflow=on
  norm : Outport
  wires:
  vector/1 -> Square/1, Divide/1
  Matrix Sum/1 -> Sqrt/1
  Divide/1 -> norm/1
  Sqrt/1 -> Divide/2
  Square/1 -> Matrix Sum/1

== system nmsRR/Supraspinal Level/Subsystem/Compute Acceleration Profiles with Minimal Jerk Approach/ Timer Phase 1/Resettable Subsystem ==
  In1 : Inport
  Enable : EnablePort  ZeroCross=off
  Out1 : Outport
  wires:
  In1/1 -> Out1/1

== system nmsRR/Supraspinal Level/Subsystem/Compute Acceleration Profiles with Minimal Jerk Approach/ Timer Phase 2/Resettable Subsystem ==
  In1 : Inport
  Enable : EnablePort  ZeroCross=off
  Out1 : Outport
  wires:
  In1/1 -> Out1/1

== system nmsRR/Supraspinal Level/Subsystem/Compute Acceleration Profiles with Minimal Jerk Approach/Minimal jerk Hip Pitch1/Enabled Subsystem ==
  In1 : Inport
  Enable : EnablePort  ZeroCross=off
  Out1 : Outport  VectorParamsAs1DForOutWhenUnconnected=off
  wires:
  In1/1 -> Out1/1

== system nmsRR/Supraspinal Level/Subsystem/Compute Acceleration Profiles with Minimal Jerk Approach/Minimal jerk Hip Pitch1/Minimal Jerk ==
  t : Inport
  a [6x1] : Inport  Port=2
  Add : Sum  Inputs=3
  Constant1 : Constant
  Constant3 : Constant  Value=2
  Demux : Demux  Outputs=6
  Divide3 : Product  Inputs=**
  Divide4 : Product  Inputs=**
  Divide5 : Product  Inputs=**
  Gain : Gain  Gain=60
  Gain1 : Gain  Gain=24
  Gain2 : Gain  Gain=6
  Math Function4 : Math  Operator=pow  SaturateOnIntegerOverflow=on
  Terminator : Terminator
  Terminator1 : Terminator
  Terminator2 : Terminator
  j(t) : Outport
  wires:
  a [6x1]/1 -> Demux/1
  Constant3/1 -> Math Function4/2
  Add/1 -> j(t)/1
  Demux/4 -> Divide3/2
  t/1 -> Divide4/1, Math Function4/1
  Demux/5 -> Divide4/2
  Demux/6 -> Divide5/2
  Demux/1 -> Terminator/1
  Demux/2 -> Terminator1/1
  Divide3/1 -> Gain2/1
  Divide4/1 -> Gain1/1
  Divide5/1 -> Gain/1
  Gain/1 -> Add/3
  Gain1/1 -> Add/2
  Gain2/1 -> Add/1
  Math Function4/1 -> Divide5/1
  Constant1/1 -> Divide3/1
  Demux/3 -> Terminator2/1

== system nmsRR/Supraspinal Level/Subsystem/Compute Acceleration Profiles with Minimal Jerk Approach/Minimal jerk Hip Pitch1/Minimal Jerk Parameters [Movellan] ==
  x0 : Inport
  dx0 : Inport  Port=2
  ddx0 : Inport  Port=3
  xT : Inport  Port=4
  dxT : Inport  Port=5
  ddxT : Inport  Port=6
  T : Inport  Port=7
  Demux : Demux  Outputs=3
  Gain : Gain  Gain=0.5
  Gain1 : Gain  Gain=3
  Gain2 : Gain  Gain=6
  Gain3 : Gain  Gain=4
  Gain4 : Gain  Gain=12
  Gain5 : Gain  Gain=5
  Gain6 : Gain  Gain=20
  Matrix Multiply : Product  Multiplication=Matrix(*)
  Minus : Sum  Inputs=+---
  Minus1 : Sum  Inputs=+--
  Minus2 : Sum  Inputs=+-
  Mux : Mux  Inputs=6
  Mux{1..4} (4 alike) : Mux  Inputs=3
  Pseudoinverse : dspinverses/Pseudoinverse  wanterr=off  SimulateUsing=Code generation
      settings: SourceProductBaseCode=DS
  T{2..5} (4 alike) : Product  Inputs=**
  b : Concatenate  NumInputs=3  Mode=Multidimensional array  ConcatenateDimension=2
  multiply : Product  Inputs=**
  multiply1 : Product  Inputs=**
  multiply2 : Product  Inputs=**
  a : Outport
  wires:
  xT/1 -> Minus/1
  Minus1/1 -> Mux4/2
  T5/1 -> Mux3/1
  multiply1/1 -> Minus1/3
  Gain5/1 -> Mux3/2
  Demux/2 -> Mux/5
  dxT/1 -> Minus1/1
  Demux/3 -> Mux/6
  b/1 -> Pseudoinverse/1
  multiply2/1 -> Minus/3
  Minus2/1 -> Mux4/3
  Gain/1 -> multiply/1, Mux/3
  multiply/1 -> Minus/4
  ddxT/1 -> Minus2/1
  Gain4/1 -> Mux2/3
  Gain6/1 -> Mux3/3
  x0/1 -> Minus/2, Mux/1
  Mux1/1 -> b/1
  Matrix Multiply/1 -> Demux/1
  ddx0/1 -> Minus2/2, multiply1/1, Gain/1
  T2/1 -> Gain1/1, Gain4/1, T3/1, multiply/2
  Gain2/1 -> Mux1/3
  Mux4/1 -> Matrix Multiply/2
  T4/1 -> Mux2/1, Gain5/1, T5/1
  Minus/1 -> Mux4/1
  Pseudoinverse/1 -> Matrix Multiply/1
  Mux2/1 -> b/2
  Gain3/1 -> Mux2/2
  Mux3/1 -> b/3
  Gain1/1 -> Mux1/2
  T/1 -> multiply2/2, multiply1/2, Gain2/1, T5/2, T4/2, T3/2, T2/2, T2/1
  Demux/1 -> Mux/4
  Mux/1 -> a/1
  T3/1 -> Gain6/1, Gain3/1, Mux1/1, T4/1
  dx0/1 -> multiply2/1, Minus1/2, Mux/2

== system nmsRR/Supraspinal Level/Subsystem/Compute Acceleration Profiles with Minimal Jerk Approach/Minimal jerk Hip Pitch2/Enabled Subsystem ==
  In1 : Inport
  Enable : EnablePort  ZeroCross=off
  Out1 : Outport  VectorParamsAs1DForOutWhenUnconnected=off
  wires:
  In1/1 -> Out1/1

== system nmsRR/Supraspinal Level/Subsystem/Compute Acceleration Profiles with Minimal Jerk Approach/Minimal jerk Hip Pitch2/Minimal Jerk ==
  t : Inport
  a [6x1] : Inport  Port=2
  Add : Sum  Inputs=3
  Constant1 : Constant
  Constant3 : Constant  Value=2
  Demux : Demux  Outputs=6
  Divide3 : Product  Inputs=**
  Divide4 : Product  Inputs=**
  Divide5 : Product  Inputs=**
  Gain : Gain  Gain=60
  Gain1 : Gain  Gain=24
  Gain2 : Gain  Gain=6
  Math Function4 : Math  Operator=pow  SaturateOnIntegerOverflow=on
  Terminator : Terminator
  Terminator1 : Terminator
  Terminator2 : Terminator
  j(t) : Outport
  wires:
  a [6x1]/1 -> Demux/1
  Constant3/1 -> Math Function4/2
  Add/1 -> j(t)/1
  Demux/4 -> Divide3/2
  t/1 -> Divide4/1, Math Function4/1
  Demux/5 -> Divide4/2
  Demux/6 -> Divide5/2
  Demux/1 -> Terminator/1
  Demux/2 -> Terminator1/1
  Divide3/1 -> Gain2/1
  Divide4/1 -> Gain1/1
  Divide5/1 -> Gain/1
  Gain/1 -> Add/3
  Gain1/1 -> Add/2
  Gain2/1 -> Add/1
  Math Function4/1 -> Divide5/1
  Constant1/1 -> Divide3/1
  Demux/3 -> Terminator2/1

== system nmsRR/Supraspinal Level/Subsystem/Compute Acceleration Profiles with Minimal Jerk Approach/Minimal jerk Hip Pitch2/Minimal Jerk Parameters [Movellan] ==
  x0 : Inport
  dx0 : Inport  Port=2
  ddx0 : Inport  Port=3
  xT : Inport  Port=4
  dxT : Inport  Port=5
  ddxT : Inport  Port=6
  T : Inport  Port=7
  Demux : Demux  Outputs=3
  Gain : Gain  Gain=0.5
  Gain1 : Gain  Gain=3
  Gain2 : Gain  Gain=6
  Gain3 : Gain  Gain=4
  Gain4 : Gain  Gain=12
  Gain5 : Gain  Gain=5
  Gain6 : Gain  Gain=20
  Matrix Multiply : Product  Multiplication=Matrix(*)
  Minus : Sum  Inputs=+---
  Minus1 : Sum  Inputs=+--
  Minus2 : Sum  Inputs=+-
  Mux : Mux  Inputs=6
  Mux{1..4} (4 alike) : Mux  Inputs=3
  Pseudoinverse : dspinverses/Pseudoinverse  wanterr=off  SimulateUsing=Code generation
      settings: SourceProductBaseCode=DS
  T{2..5} (4 alike) : Product  Inputs=**
  b : Concatenate  NumInputs=3  Mode=Multidimensional array  ConcatenateDimension=2
  multiply : Product  Inputs=**
  multiply1 : Product  Inputs=**
  multiply2 : Product  Inputs=**
  a : Outport
  wires:
  xT/1 -> Minus/1
  Minus1/1 -> Mux4/2
  T5/1 -> Mux3/1
  multiply1/1 -> Minus1/3
  Gain5/1 -> Mux3/2
  Demux/2 -> Mux/5
  dxT/1 -> Minus1/1
  Demux/3 -> Mux/6
  b/1 -> Pseudoinverse/1
  multiply2/1 -> Minus/3
  Minus2/1 -> Mux4/3
  Gain/1 -> multiply/1, Mux/3
  multiply/1 -> Minus/4
  ddxT/1 -> Minus2/1
  Gain4/1 -> Mux2/3
  Gain6/1 -> Mux3/3
  x0/1 -> Minus/2, Mux/1
  Mux1/1 -> b/1
  Matrix Multiply/1 -> Demux/1
  ddx0/1 -> Minus2/2, multiply1/1, Gain/1
  T2/1 -> Gain1/1, Gain4/1, T3/1, multiply/2
  Gain2/1 -> Mux1/3
  Mux4/1 -> Matrix Multiply/2
  T4/1 -> Mux2/1, Gain5/1, T5/1
  Minus/1 -> Mux4/1
  Pseudoinverse/1 -> Matrix Multiply/1
  Mux2/1 -> b/2
  Gain3/1 -> Mux2/2
  Mux3/1 -> b/3
  Gain1/1 -> Mux1/2
  T/1 -> multiply2/2, multiply1/2, Gain2/1, T5/2, T4/2, T3/2, T2/2, T2/1
  Demux/1 -> Mux/4
  Mux/1 -> a/1
  T3/1 -> Gain6/1, Gain3/1, Mux1/1, T4/1
  dx0/1 -> multiply2/1, Minus1/2, Mux/2

== system nmsRR/Supraspinal Level/Subsystem/Compute Acceleration Profiles with Minimal Jerk Approach/Minimal jerk Hip Pitch3/Enabled Subsystem ==
  In1 : Inport
  Enable : EnablePort  ZeroCross=off
  Out1 : Outport  VectorParamsAs1DForOutWhenUnconnected=off
  wires:
  In1/1 -> Out1/1

== system nmsRR/Supraspinal Level/Subsystem/Compute Acceleration Profiles with Minimal Jerk Approach/Minimal jerk Hip Pitch3/Minimal Jerk ==
  t : Inport
  a [6x1] : Inport  Port=2
  Add : Sum  Inputs=3
  Constant1 : Constant
  Constant3 : Constant  Value=2
  Demux : Demux  Outputs=6
  Divide3 : Product  Inputs=**
  Divide4 : Product  Inputs=**
  Divide5 : Product  Inputs=**
  Gain : Gain  Gain=60
  Gain1 : Gain  Gain=24
  Gain2 : Gain  Gain=6
  Math Function4 : Math  Operator=pow  SaturateOnIntegerOverflow=on
  Terminator : Terminator
  Terminator1 : Terminator
  Terminator2 : Terminator
  j(t) : Outport
  wires:
  a [6x1]/1 -> Demux/1
  Constant3/1 -> Math Function4/2
  Add/1 -> j(t)/1
  Demux/4 -> Divide3/2
  t/1 -> Divide4/1, Math Function4/1
  Demux/5 -> Divide4/2
  Demux/6 -> Divide5/2
  Demux/1 -> Terminator/1
  Demux/2 -> Terminator1/1
  Divide3/1 -> Gain2/1
  Divide4/1 -> Gain1/1
  Divide5/1 -> Gain/1
  Gain/1 -> Add/3
  Gain1/1 -> Add/2
  Gain2/1 -> Add/1
  Math Function4/1 -> Divide5/1
  Constant1/1 -> Divide3/1
  Demux/3 -> Terminator2/1

== system nmsRR/Supraspinal Level/Subsystem/Compute Acceleration Profiles with Minimal Jerk Approach/Minimal jerk Hip Pitch3/Minimal Jerk Parameters [Movellan] ==
  x0 : Inport
  dx0 : Inport  Port=2
  ddx0 : Inport  Port=3
  xT : Inport  Port=4
  dxT : Inport  Port=5
  ddxT : Inport  Port=6
  T : Inport  Port=7
  Demux : Demux  Outputs=3
  Gain : Gain  Gain=0.5
  Gain1 : Gain  Gain=3
  Gain2 : Gain  Gain=6
  Gain3 : Gain  Gain=4
  Gain4 : Gain  Gain=12
  Gain5 : Gain  Gain=5
  Gain6 : Gain  Gain=20
  Matrix Multiply : Product  Multiplication=Matrix(*)
  Minus : Sum  Inputs=+---
  Minus1 : Sum  Inputs=+--
  Minus2 : Sum  Inputs=+-
  Mux : Mux  Inputs=6
  Mux{1..4} (4 alike) : Mux  Inputs=3
  Pseudoinverse : dspinverses/Pseudoinverse  wanterr=off  SimulateUsing=Code generation
      settings: SourceProductBaseCode=DS
  T{2..5} (4 alike) : Product  Inputs=**
  b : Concatenate  NumInputs=3  Mode=Multidimensional array  ConcatenateDimension=2
  multiply : Product  Inputs=**
  multiply1 : Product  Inputs=**
  multiply2 : Product  Inputs=**
  a : Outport
  wires:
  xT/1 -> Minus/1
  Minus1/1 -> Mux4/2
  T5/1 -> Mux3/1
  multiply1/1 -> Minus1/3
  Gain5/1 -> Mux3/2
  Demux/2 -> Mux/5
  dxT/1 -> Minus1/1
  Demux/3 -> Mux/6
  b/1 -> Pseudoinverse/1
  multiply2/1 -> Minus/3
  Minus2/1 -> Mux4/3
  Gain/1 -> multiply/1, Mux/3
  multiply/1 -> Minus/4
  ddxT/1 -> Minus2/1
  Gain4/1 -> Mux2/3
  Gain6/1 -> Mux3/3
  x0/1 -> Minus/2, Mux/1
  Mux1/1 -> b/1
  Matrix Multiply/1 -> Demux/1
  ddx0/1 -> Minus2/2, multiply1/1, Gain/1
  T2/1 -> Gain1/1, Gain4/1, T3/1, multiply/2
  Gain2/1 -> Mux1/3
  Mux4/1 -> Matrix Multiply/2
  T4/1 -> Mux2/1, Gain5/1, T5/1
  Minus/1 -> Mux4/1
  Pseudoinverse/1 -> Matrix Multiply/1
  Mux2/1 -> b/2
  Gain3/1 -> Mux2/2
  Mux3/1 -> b/3
  Gain1/1 -> Mux1/2
  T/1 -> multiply2/2, multiply1/2, Gain2/1, T5/2, T4/2, T3/2, T2/2, T2/1
  Demux/1 -> Mux/4
  Mux/1 -> a/1
  T3/1 -> Gain6/1, Gain3/1, Mux1/1, T4/1
  dx0/1 -> multiply2/1, Minus1/2, Mux/2

== system nmsRR/Supraspinal Level/Subsystem/Compute Acceleration Profiles with Minimal Jerk Approach/Minimal jerk Hip Pitch4/Enabled Subsystem ==
  In1 : Inport
  Enable : EnablePort  ZeroCross=off
  Out1 : Outport  VectorParamsAs1DForOutWhenUnconnected=off
  wires:
  In1/1 -> Out1/1

== system nmsRR/Supraspinal Level/Subsystem/Compute Acceleration Profiles with Minimal Jerk Approach/Minimal jerk Hip Pitch4/Minimal Jerk ==
  t : Inport
  a [6x1] : Inport  Port=2
  Add : Sum  Inputs=3
  Constant1 : Constant
  Constant3 : Constant  Value=2
  Demux : Demux  Outputs=6
  Divide3 : Product  Inputs=**
  Divide4 : Product  Inputs=**
  Divide5 : Product  Inputs=**
  Gain : Gain  Gain=60
  Gain1 : Gain  Gain=24
  Gain2 : Gain  Gain=6
  Math Function4 : Math  Operator=pow  SaturateOnIntegerOverflow=on
  Terminator : Terminator
  Terminator1 : Terminator
  Terminator2 : Terminator
  j(t) : Outport
  wires:
  a [6x1]/1 -> Demux/1
  Constant3/1 -> Math Function4/2
  Add/1 -> j(t)/1
  Demux/4 -> Divide3/2
  t/1 -> Divide4/1, Math Function4/1
  Demux/5 -> Divide4/2
  Demux/6 -> Divide5/2
  Demux/1 -> Terminator/1
  Demux/2 -> Terminator1/1
  Divide3/1 -> Gain2/1
  Divide4/1 -> Gain1/1
  Divide5/1 -> Gain/1
  Gain/1 -> Add/3
  Gain1/1 -> Add/2
  Gain2/1 -> Add/1
  Math Function4/1 -> Divide5/1
  Constant1/1 -> Divide3/1
  Demux/3 -> Terminator2/1
